simulink model "WF_offshore"  (R2024a)
settings: Solver=VariableStepAuto  StartTime=0  StopTime=1  RelTol=1e-3
values from neighbouring files (symbols this model uses):
  WF = calculate_WF(WF)    [WF_parameter_variation.m]
undefined symbols (not defined in the file or in its folder): L, Lg, R
libraries: spsSeriesRLCBranchLib x24, spsGroundLib x11, simulink_extras x8, spsThreePhaseVIMeasurementLib x6, spsControlledVoltageSourceLib x6, spsIdealSwitchLib x6, simulink x4, spsVariableInductorLib x3, spsThreePhaseSeriesRLCBranchLib x2, spsThreePhaseTransformerTwoWindingsLib x2, powerlib_extras x1, spspowerguiLib x1
(part 1 of 2)
settings Model: Creator=andrsmit  LastModifiedBy=andrsmit
settings DataIOCC: InitialState=op.xFinal  SaveFinalState=on  SaveOperatingPoint=on

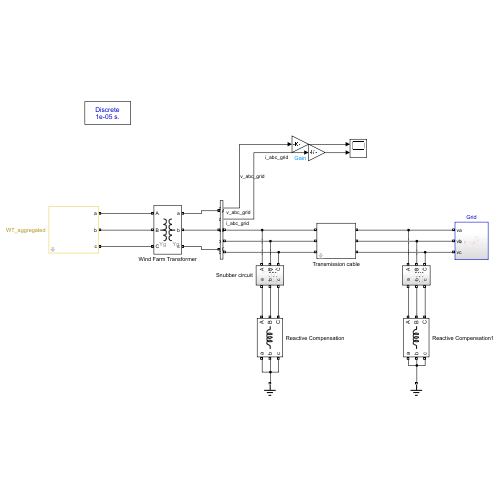
[thumbnail: Simulink's stored preview of the top-level diagram]
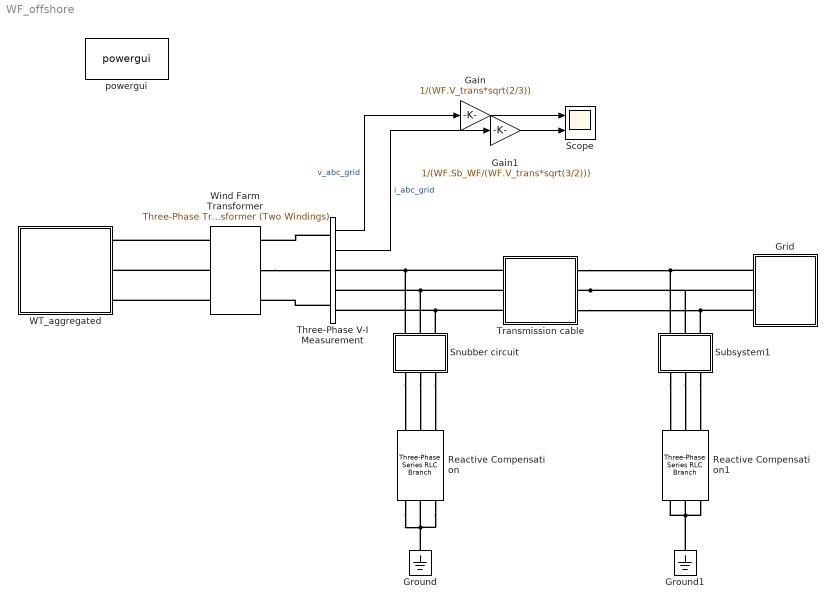
== system WF_offshore ==
  Gain : Gain  Gain=1/(WF.V_trans*sqrt(2/3))
  Gain1 : Gain  Gain=1/(WF.Sb_WF/(WF.V_trans*sqrt(3/2)))
  Grid : Subsystem
  Ground : spsGroundLib/Ground  LConnTagsString=a
  Ground1 : spsGroundLib/Ground  LConnTagsString=a
  Reactive Compensation : spsThreePhaseSeriesRLCBranchLib/Three-Phase Series RLC Branch  LConnTagsString=A|B|C  RConnTagsString=A|B|C  BranchType=L  Resistance=100  Inductance=WF.L_comp  Capacitance=1e-6  Measurements=None
  Reactive Compensation1 : spsThreePhaseSeriesRLCBranchLib/Three-Phase Series RLC Branch  LConnTagsString=A|B|C  RConnTagsString=A|B|C  BranchType=L  Resistance=100  Inductance=WF.L_comp  Capacitance=1e-6  Measurements=None
  Scope : Scope  NumInputPorts=2
  Snubber circuit : Subsystem
  Subsystem1 : Subsystem
  Three-Phase V-I Measurement : spsThreePhaseVIMeasurementLib/Three-Phase V-I Measurement  VoltageMeasurement=phase-to-ground  SetLabelV=off  LabelV=Vabc  Vpu=off  VpuLL=off  CurrentMeasurement=yes  SetLabelI=off  LabelI=Iabc  Ipu=off  Pbase=100e6  Vbase=500e3  OutputType=Complex  PhasorSimulation=off  PSBequivalent=0
  Transmission cable : Subsystem  mask{D=WF.Trans.D_C, r=WF.Trans.r_c_eff, l=WF.Trans.l_c_eff, c=WF.Trans.c_c_eff}
      mask prompts: D "Distance (km)"; r "Resistance/km (Ohms/km)"; l "Inductance/km (H/km)"; c "Capacitance/km (F/km)"
      mask DialogControl DescTextVar Prompt: Single PI-line cable model, with no coupling/connection between phases
  WT_aggregated : Subsystem  mask{cvtr=WF.WT.cvtr_agg}
      mask prompts: cvtr "converter name"
  Wind Farm Transformer : spsThreePhaseTransformerTwoWindingsLib/Three-Phase Transformer (Two Windings)  Winding1Connection=Yg  Winding2Connection=Yg  CoreType=Three single-phase transformers  SetSaturation=off  Hysteresis=off  DataFile='hysteresis'  SetInitialFlux=off  Measurements=None  UNITS=pu  NominalPower=[WF.Sb_WF , WF.f1]  Winding1=[WF.V_coll , WF.r_tf/2, WF.l_tf/2]  Winding2=[WF.V_trans, WF.r_tf/2, WF.l_tf/2]  Rm=5000  Lm=0  L0=0.5  Saturation=[ 0,0 ; 0.0024,1.2 ; 1.0,1.52 ]  InitialFluxes=[ 0.8 , -0.8 , 0.7 ]  BreakLoop=off  DiscreteSolver=Trapezoidal iterative  DataType=off  TransfoNumber=1
  powergui : spspowerguiLib/powergui  Priority=2  SimulationMode=Discrete  SampleTime=WF.WT.cvtr_agg.parameters.Ts  frequency=60  Iterations=50  frequencyindice=0  Pbase=100e6  ErrMax=0.0001  UnitsV=kV  UnitsW=MW  buscounter=0  FunctionMessages=off  echomessages=off  EnableUseOfTLC=off  CurrentSourceSwitches=off  DisableSnubberDevices=off  DisableRonSwitches=off  DisableVfSwitches=off  DisplayEquations=off  AutomaticDiscreteSolvers=off  SolverType=Tustin  Interpol=off  ExternalGateDelay=off  methode=off  Ts=0  x0status=blocks  SPID=off  SwTol=0  HookPort=off  NonlinearTolerance=1e-4  nMaxIteration=100  ContinueOnMaxIteration=off  RestoreLinks=warning  ResistiveCurrentMeasurement=off  Frange=logspace(0,3,50)  Ylog=off  Xlog=off  ShowGrid=off  save=off  variable=ZData  structure=0  ZoomFFT=on  StartTime=0.0  cycles=1  DisplayStyle=1  fundamental=60  FreqAxis=off  MaxFrequency=1000  frequencyindicesteady=1  RmsSteady=1  display=off
  wires:
  Three-Phase V-I Measurement/1 -> Gain/1  "v_abc_grid"
  Three-Phase V-I Measurement/2 -> Gain1/1  "i_abc_grid"
  Gain1/1 -> Scope/2
  Gain/1 -> Scope/1
  connections:
  Three-Phase V-I Measurement/LConn1 -- Wind Farm Transformer/RConn1
  Wind Farm Transformer/RConn2 -- Three-Phase V-I Measurement/LConn2
  Three-Phase V-I Measurement/LConn3 -- Wind Farm Transformer/RConn3
  Transmission cable/RConn1 -- Grid/RConn1 -- Subsystem1/LConn1
  Transmission cable/RConn2 -- Grid/RConn2 -- Subsystem1/LConn2
  Transmission cable/LConn3 -- Snubber circuit/LConn3 -- Three-Phase V-I Measurement/RConn3
  Ground/LConn1 -- Reactive Compensation/RConn1 -- Reactive Compensation/RConn3 -- Reactive Compensation/RConn2
  Reactive Compensation1/RConn3 -- Reactive Compensation1/RConn1 -- Ground1/LConn1 -- Reactive Compensation1/RConn2
  Transmission cable/RConn3 -- Grid/RConn3 -- Subsystem1/LConn3
  Snubber circuit/RConn2 -- Reactive Compensation/LConn2
  Snubber circuit/RConn1 -- Reactive Compensation/LConn1
  Transmission cable/LConn2 -- Snubber circuit/LConn2 -- Three-Phase V-I Measurement/RConn2
  Snubber circuit/RConn3 -- Reactive Compensation/LConn3
  Transmission cable/LConn1 -- Three-Phase V-I Measurement/RConn1 -- Snubber circuit/LConn1
  Subsystem1/RConn3 -- Reactive Compensation1/LConn3
  Subsystem1/RConn1 -- Reactive Compensation1/LConn1
  Subsystem1/RConn2 -- Reactive Compensation1/LConn2
  Wind Farm Transformer/LConn3 -- WT_aggregated/RConn3
  Wind Farm Transformer/LConn2 -- WT_aggregated/RConn2
  Wind Farm Transformer/LConn1 -- WT_aggregated/RConn1

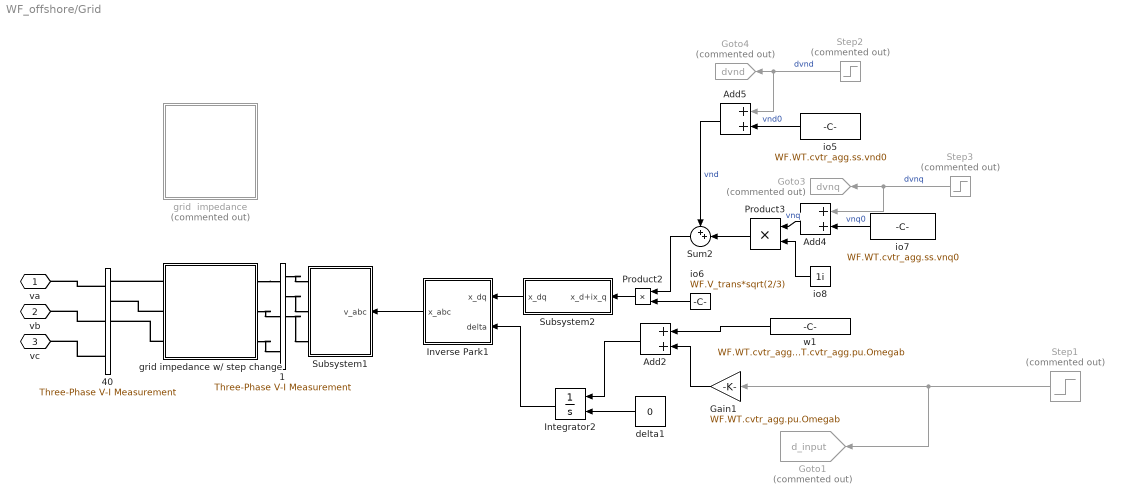
== system WF_offshore/Grid ==
  1 : spsThreePhaseVIMeasurementLib/Three-Phase V-I Measurement  VoltageMeasurement=phase-to-ground  SetLabelV=off  LabelV=Vabc_1  Vpu=off  VpuLL=off  CurrentMeasurement=yes  SetLabelI=off  LabelI=Iabc_1  Ipu=off  Pbase=100e6  Vbase=Bus(1,2)*1e3  OutputType=Complex  PhasorSimulation=off  PSBequivalent=0
  40 : spsThreePhaseVIMeasurementLib/Three-Phase V-I Measurement  VoltageMeasurement=phase-to-ground  SetLabelV=off  LabelV=Vabc_1  Vpu=off  VpuLL=off  CurrentMeasurement=yes  SetLabelI=off  LabelI=Iabc_1  Ipu=off  Pbase=100e6  Vbase=Bus(1,2)*1e3  OutputType=Complex  PhasorSimulation=off  PSBequivalent=0
  Add2 : Sum
  Add4 : Sum
  Add5 : Sum
  Gain1 : Gain  Gain=WF.WT.cvtr_agg.pu.Omegab
  Goto1 : Goto  Commented=on  GotoTag=d_input  TagVisibility=global
  Goto3 : Goto  Commented=on  GotoTag=dvnq  TagVisibility=global
  Goto4 : Goto  Commented=on  GotoTag=dvnd  TagVisibility=global
  Integrator2 : Integrator  InitialConditionSource=external
  Inverse Park1 : Subsystem
  Product2 : Product
  Product3 : Product
  Step1 : Step  Commented=on  Time=0.1  After=1e-4  SampleTime=0
  Step2 : Step  Commented=on  Time=0.1  After=0.01  SampleTime=0
  Step3 : Step  Commented=on  Time=0.1  After=0.01  SampleTime=0
  Subsystem1 : Subsystem
  Subsystem2 : Subsystem
  Sum2 : Sum  Inputs=++|
  delta1 : Constant  Value=0
  grid  impedance : Subsystem  Commented=on
  grid impedance w/ step change : Subsystem
  io5 : Constant  Value=WF.WT.cvtr_agg.ss.vnd0
  io6 : Constant  Value=WF.V_trans*sqrt(2/3)
  io7 : Constant  Value=WF.WT.cvtr_agg.ss.vnq0
  io8 : Constant  Value=1i
  w1 : Constant  Value=WF.WT.cvtr_agg.parameters.Omegag*WF.WT.cvtr_agg.pu.Omegab
  va : PMIOPort  Side=Right
  vb : PMIOPort  Port=2  Side=Right
  vc : PMIOPort  Port=3  Side=Right
  wires:
  Integrator2/1 -> Inverse Park1/2(delta)
  io5/1 -> Add5/2  "vnd0"
  Add4/1 -> Product3/1  "vnq"
  Subsystem2/1(x_dq) -> Inverse Park1/1(x_dq)
  Add2/1 -> Integrator2/1
  Inverse Park1/1(x_abc) -> Subsystem1/1(v_abc)
  Sum2/1 -> Product2/1
  io7/1 -> Add4/2  "vnq0"
  w1/1 -> Add2/1
  Step1/1 -> Goto1/1, Gain1/1
  Step3/1 -> Goto3/1, Add4/1  "dvnq"
  Add5/1 -> Sum2/1  "vnd"
  delta1/1 -> Integrator2/2
  Step2/1 -> Add5/1, Goto4/1  "dvnd"
  Product2/1 -> Subsystem2/1(x_d+ix_q)
  io8/1 -> Product3/2
  io6/1 -> Product2/2
  Product3/1 -> Sum2/2
  Gain1/1 -> Add2/2
  connections:
  40/LConn1 -- vc/RConn1
  40/LConn2 -- vb/RConn1
  40/LConn3 -- va/RConn1
  grid impedance w/ step change/LConn1 -- 40/RConn3
  grid impedance w/ step change/LConn2 -- 40/RConn2
  grid impedance w/ step change/LConn3 -- 40/RConn1
  grid impedance w/ step change/RConn1 -- 1/LConn3
  grid impedance w/ step change/RConn2 -- 1/LConn2
  grid impedance w/ step change/RConn3 -- 1/LConn1
  1/RConn3 -- Subsystem1/RConn1
  1/RConn2 -- Subsystem1/RConn2
  1/RConn1 -- Subsystem1/RConn3

== system WF_offshore/Snubber circuit ==
  Ideal Switch : spsIdealSwitchLib/Ideal Switch  Ron=WF.R_comp  Lon=0  IC=0  Rs=WF.r_diss*WF.Imp.Z_b_G  Cs=inf  Measurements=off
  Ideal Switch1 : spsIdealSwitchLib/Ideal Switch  Ron=WF.R_comp  Lon=0  IC=0  Rs=WF.r_diss*WF.Imp.Z_b_G  Cs=inf  Measurements=off
  Ideal Switch2 : spsIdealSwitchLib/Ideal Switch  Ron=WF.R_comp  Lon=0  IC=0  Rs=WF.r_diss*WF.Imp.Z_b_G  Cs=inf  Measurements=off
  Step : Step  Time=0.5  SampleTime=0
  " A" : PMIOPort  Side=Left
  " B" : PMIOPort  Port=2  Side=Left
  " C" : PMIOPort  Port=3  Side=Left
  "  a" : PMIOPort  Port=4  Side=Right
  "  b" : PMIOPort  Port=5  Side=Right
  "  c" : PMIOPort  Port=6  Side=Right
  wires:
  Step/1 -> Ideal Switch2/1, Ideal Switch1/1, Ideal Switch/1
  connections:
  "  a"/RConn1 -- Ideal Switch/RConn1
  Ideal Switch2/LConn1 -- " C"/RConn1
  Ideal Switch2/RConn1 -- "  c"/RConn1
  " A"/RConn1 -- Ideal Switch/LConn1
  Ideal Switch1/RConn1 -- "  b"/RConn1
  Ideal Switch1/LConn1 -- " B"/RConn1

== system WF_offshore/Subsystem1 ==
  Ideal Switch : spsIdealSwitchLib/Ideal Switch  Ron=WF.R_comp  Lon=0  IC=0  Rs=WF.r_diss*WF.Imp.Z_b_G  Cs=inf  Measurements=off
  Ideal Switch1 : spsIdealSwitchLib/Ideal Switch  Ron=WF.R_comp  Lon=0  IC=0  Rs=WF.r_diss*WF.Imp.Z_b_G  Cs=inf  Measurements=off
  Ideal Switch2 : spsIdealSwitchLib/Ideal Switch  Ron=WF.R_comp  Lon=0  IC=0  Rs=WF.r_diss*WF.Imp.Z_b_G  Cs=inf  Measurements=off
  Step : Step  Time=0.5  SampleTime=0
  " A" : PMIOPort  Side=Left
  " B" : PMIOPort  Port=2  Side=Left
  " C" : PMIOPort  Port=3  Side=Left
  "  a" : PMIOPort  Port=4  Side=Right
  "  b" : PMIOPort  Port=5  Side=Right
  "  c" : PMIOPort  Port=6  Side=Right
  wires:
  Step/1 -> Ideal Switch2/1, Ideal Switch1/1, Ideal Switch/1
  connections:
  "  a"/RConn1 -- Ideal Switch/RConn1
  Ideal Switch2/LConn1 -- " C"/RConn1
  Ideal Switch2/RConn1 -- "  c"/RConn1
  " A"/RConn1 -- Ideal Switch/LConn1
  Ideal Switch1/RConn1 -- "  b"/RConn1
  Ideal Switch1/LConn1 -- " B"/RConn1

== system WF_offshore/Transmission cable ==
  Subsystem : Subsystem
  Subsystem1 : Subsystem
  Subsystem2 : Subsystem
  A : PMIOPort  Side=Left
  a : PMIOPort  Port=2  Side=Right
  B : PMIOPort  Port=3  Side=Left
  b : PMIOPort  Port=4  Side=Right
  C : PMIOPort  Port=5  Side=Left
  c : PMIOPort  Port=6  Side=Right
  connections:
  Subsystem/RConn1 -- a/RConn1
  Subsystem/LConn1 -- A/RConn1
  Subsystem1/LConn1 -- B/RConn1
  Subsystem2/RConn1 -- c/RConn1
  Subsystem1/RConn1 -- b/RConn1
  Subsystem2/LConn1 -- C/RConn1

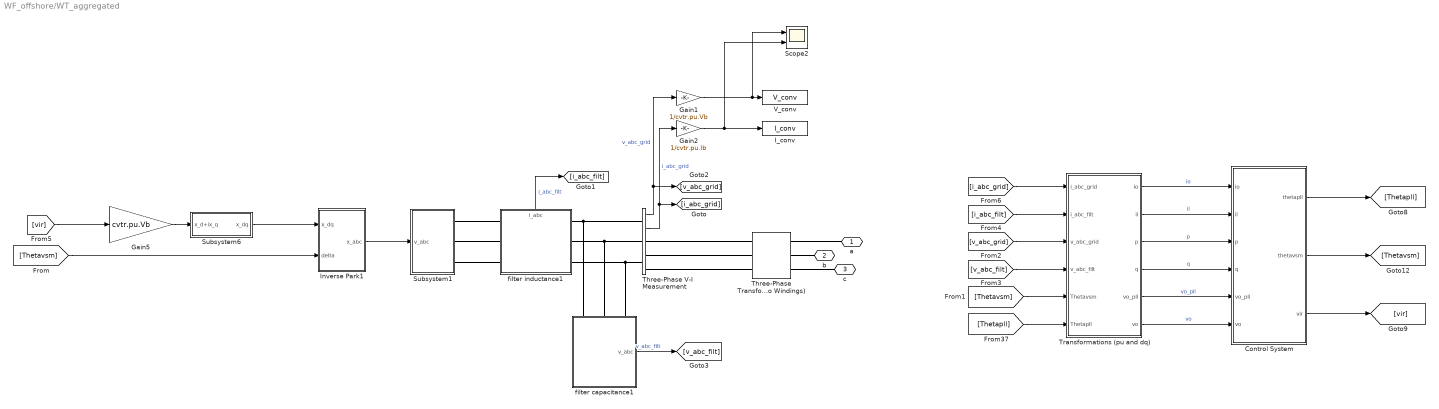
== system WF_offshore/WT_aggregated ==
  Control System : Subsystem  mask{Ts_control=cvtr.parameters.T_cont}
      mask prompts: Ts_control "Sample Time"
  Gain1 : Gain  Gain=1/cvtr.pu.Vb
  Gain2 : Gain  Gain=1/cvtr.pu.Ib
  Gain5 : Gain  Gain=cvtr.pu.Vb
  I_conv : ToWorkspace  VariableName=I_conv  SaveFormat=Structure With Time  SampleTime=-1
      settings: MaxDataPoints=1000000
  Inverse Park1 : Subsystem
  Scope2 : Scope  NumInputPorts=2
  Subsystem1 : Subsystem
  Subsystem6 : Subsystem
  Three-Phase Transformer (Two Windings) : spsThreePhaseTransformerTwoWindingsLib/Three-Phase Transformer (Two Windings)  Winding1Connection=Yg  Winding2Connection=Yg  CoreType=Three single-phase transformers  SetSaturation=off  Hysteresis=off  DataFile='hysteresis'  SetInitialFlux=off  Measurements=None  UNITS=pu  NominalPower=[WF.Sb_WF , WF.f1 ]  Winding1=[WF.WT.V_wt ,WF.WT.r_tf/2 , WF.WT.l_tf/2]  Winding2=[WF.V_coll , WF.WT.r_tf/2, WF.WT.l_tf/2]  Rm=5000  Lm=0  L0=0.5  Saturation=[ 0,0 ; 0.0024,1.2 ; 1.0,1.52 ]  InitialFluxes=[ 0.8 , -0.8 , 0.7 ]  BreakLoop=off  DiscreteSolver=Trapezoidal iterative  DataType=off  TransfoNumber=1
  Three-Phase V-I Measurement : spsThreePhaseVIMeasurementLib/Three-Phase V-I Measurement  VoltageMeasurement=phase-to-ground  SetLabelV=off  LabelV=Vabc  Vpu=off  VpuLL=off  CurrentMeasurement=yes  SetLabelI=off  LabelI=Iabc  Ipu=off  Pbase=100e6  Vbase=500e3  OutputType=Complex  PhasorSimulation=off  PSBequivalent=0
  Transformations (pu and dq) : Subsystem
  V_conv : ToWorkspace  VariableName=V_conv  SaveFormat=Structure With Time  SampleTime=-1
      settings: MaxDataPoints=1000000
  filter capacitance1 : Subsystem
      settings: PortSchema="{\"entries\":[{\"content\":{\"sides\":[{\"content\":{\"connectorIds\":[\"LConn1\",\"LConn2\",\"LConn3\"]},\"type\":\"ConnectorPlacement.EquallySpacedRectSide\",\"uuid\":\"e81be3d5-6303-4565-8ca3-afc618f21d70\"},{\"content\":{\"connectorIds\":[],\"side\":\"RIGHT\"},\"type\":\"ConnectorPlacement.EquallySpacedRectSide\",\"uuid\":\"458d9030-e614-487d-87de-3e53be7c7da4\"},{\"content\":{\"connectorIds\":[],\"side\":\"TOP\"},\"type\":\"ConnectorPlacement.EquallySpacedRectSide\",\"uuid\":\"a29d66a0-f095-498d-bb9b-96c7f47699d3\"},{\"content\":{\"connectorIds\":[\"Out1\"],\"side\":\"BOTTOM\"},\"type\":\"ConnectorPlacement.EquallySpacedRectSide\",\"uuid\":\"afc68874-c098-43f5-9b37-53a3b484513b\"}]},\"type\":\"ConnectorPlacement.EquallySpacedConnector\",\"uuid\":\"37f495dd-1c12-4bb8-af72-7ef46bbd951c\"}],\"packageUris\":[\"http://schema.mathworks.com/mf0/Connector/R2020b\"],\"version\":\"1.0\"}"
  filter inductance1 : Subsystem
      settings: PortSchema="{\"entries\":[{\"content\":{\"sides\":[{\"content\":{\"connectorIds\":[\"LConn1\",\"LConn2\",\"LConn3\"]},\"type\":\"ConnectorPlacement.EquallySpacedRectSide\",\"uuid\":\"d3d60048-9578-4fa3-8d11-9c8a66a4b1f9\"},{\"content\":{\"connectorIds\":[\"RConn1\",\"RConn2\",\"RConn3\"],\"side\":\"RIGHT\"},\"type\":\"ConnectorPlacement.EquallySpacedRectSide\",\"uuid\":\"184a2c1d-36ab-46d1-99e4-db01aa31ec94\"},{\"content\":{\"connectorIds\":[\"Out1\"],\"side\":\"TOP\"},\"type\":\"ConnectorPlacement.EquallySpacedRectSide\",\"uuid\":\"db651021-9d7f-4124-8d21-ede853163467\"}]},\"type\":\"ConnectorPlacement.EquallySpacedConnector\",\"uuid\":\"723d0964-19fd-4dbe-91e3-e4ea0bb1cca9\"}],\"packageUris\":[\"http://schema.mathworks.com/mf0/Connector/R2020b\"],\"version\":\"1.0\"}"
  a : PMIOPort  Side=Right
  b : PMIOPort  Port=2  Side=Right
  c : PMIOPort  Port=3  Side=Right
  wires:
  Control System/2(thetavsm) -> [Thetavsm]
  Control System/3(vir) -> [vir]
  Control System/1(thetapll) -> [Thetapll]
  Transformations (pu and dq)/2(il) -> Control System/2(il)  "il"
  Transformations (pu and dq)/1(io) -> Control System/1(io)  "io"
  Transformations (pu and dq)/3(p) -> Control System/3(p)  "p"
  Transformations (pu and dq)/4(q) -> Control System/4(q)  "q"
  Transformations (pu and dq)/5(vo_pll) -> Control System/5(vo_pll)  "vo_pll"
  Transformations (pu and dq)/6(vo) -> Control System/6(vo)  "vo"
  [Thetavsm] -> Transformations (pu and dq)/5(Thetavsm)
  [Thetapll] -> Transformations (pu and dq)/6(Thetapll)
  [vir] -> Gain5/1
  Subsystem6/1(x_dq) -> Inverse Park1/1(x_dq)
  Gain5/1 -> Subsystem6/1(x_d+ix_q)
  Three-Phase V-I Measurement/2 -> Gain2/1, [i_abc_grid]  "i_abc_grid"
  Inverse Park1/1(x_abc) -> Subsystem1/1(v_abc)
  Three-Phase V-I Measurement/1 -> Gain1/1, [v_abc_grid]  "v_abc_grid"
  [Thetavsm] -> Inverse Park1/2(delta)
  filter capacitance1/1(v_abc) -> [v_abc_filt]  "v_abc_filt"
  filter inductance1/1(i_abc) -> [i_abc_filt]  "i_abc_filt"
  [v_abc_grid] -> Transformations (pu and dq)/3(v_abc_grid)
  [v_abc_filt] -> Transformations (pu and dq)/4(v_abc_filt)
  [i_abc_filt] -> Transformations (pu and dq)/2(i_abc_filt)
  [i_abc_grid] -> Transformations (pu and dq)/1(i_abc_grid)
  Gain1/1 -> Scope2/1, V_conv/1
  Gain2/1 -> Scope2/2, I_conv/1
  connections:
  filter inductance1/RConn3 -- filter capacitance1/LConn3 -- Three-Phase V-I Measurement/LConn3
  filter inductance1/RConn1 -- filter capacitance1/LConn1 -- Three-Phase V-I Measurement/LConn1
  filter inductance1/RConn2 -- filter capacitance1/LConn2 -- Three-Phase V-I Measurement/LConn2
  Subsystem1/RConn1 -- filter inductance1/LConn1
  Subsystem1/RConn2 -- filter inductance1/LConn2
  Subsystem1/RConn3 -- filter inductance1/LConn3
  Three-Phase Transformer (Two Windings)/RConn1 -- a/RConn1
  Three-Phase Transformer (Two Windings)/RConn2 -- b/RConn1
  Three-Phase Transformer (Two Windings)/RConn3 -- c/RConn1
  Three-Phase Transformer (Two Windings)/LConn1 -- Three-Phase V-I Measurement/RConn1
  Three-Phase Transformer (Two Windings)/LConn2 -- Three-Phase V-I Measurement/RConn2
  Three-Phase Transformer (Two Windings)/LConn3 -- Three-Phase V-I Measurement/RConn3

== system WF_offshore/Grid/Inverse Park1 ==
  x_dq : Inport
  delta : Inport  Port=2
  Demux1 : Demux  Outputs=2
  Fcn : Fcn  Expr=cos(u(3))*u(1)-sin(u(3))*u(2)
  Fcn1 : Fcn  Expr=cos(u(3)-2/3*pi)*u(1)-sin(u(3)-2/3*pi)*u(2)
  Fcn2 : Fcn  Expr=cos(u(3)+2/3*pi)*u(1)-sin(u(3)+2/3*pi)*u(2)
  Mux : Mux  Inputs=3
  Mux1 : Mux  Inputs=3
  x_abc : Outport
  wires:
  Mux1/1 -> x_abc/1
  Mux/1 -> Fcn1/1, Fcn2/1, Fcn/1
  delta/1 -> Mux/3
  x_dq/1 -> Demux1/1
  Demux1/2 -> Mux/2
  Demux1/1 -> Mux/1
  Fcn/1 -> Mux1/1
  Fcn1/1 -> Mux1/2
  Fcn2/1 -> Mux1/3

== system WF_offshore/Grid/Subsystem1 ==
  v_abc : Inport
  Controlled Voltage Source : spsControlledVoltageSourceLib/Controlled Voltage Source  Initialize=on  Source_Type=AC  Amplitude=0  Phase=0  Frequency=0  Measurements=None
  Controlled Voltage Source1 : spsControlledVoltageSourceLib/Controlled Voltage Source  Initialize=on  Source_Type=AC  Amplitude=0  Phase=0  Frequency=0  Measurements=None
  Controlled Voltage Source2 : spsControlledVoltageSourceLib/Controlled Voltage Source  Initialize=on  Source_Type=AC  Amplitude=0  Phase=0  Frequency=0  Measurements=None
  Demux : Demux  Outputs=3
  Ground1 : spsGroundLib/Ground  LConnTagsString=a
  va : PMIOPort  Side=Right
  vb : PMIOPort  Port=2  Side=Right
  vc : PMIOPort  Port=3  Side=Right
  wires:
  Demux/1 -> Controlled Voltage Source/1
  Demux/2 -> Controlled Voltage Source1/1
  Demux/3 -> Controlled Voltage Source2/1
  v_abc/1 -> Demux/1
  connections:
  Controlled Voltage Source2/LConn1 -- Ground1/LConn1 -- Controlled Voltage Source1/LConn1 -- Controlled Voltage Source/LConn1
  va/RConn1 -- Controlled Voltage Source/RConn1
  vb/RConn1 -- Controlled Voltage Source1/RConn1
  vc/RConn1 -- Controlled Voltage Source2/RConn1

== system WF_offshore/Grid/Subsystem2 ==
  x_d+ix_q : Inport
  Complex to Real-Imag2 : ComplexToRealImag
  Mux : Mux  Inputs=2
  x_dq : Outport
  wires:
  Complex to Real-Imag2/1 -> Mux/1
  Complex to Real-Imag2/2 -> Mux/2
  Mux/1 -> x_dq/1
  x_d+ix_q/1 -> Complex to Real-Imag2/1

== system WF_offshore/Grid/grid  impedance ==
  Series RLC Branch : spsSeriesRLCBranchLib/Series RLC Branch  LConnTagsString=__new0  RConnTagsString=__new0  BranchType=RL  Resistance=(WF.Trans.rg)*WF.Imp.Z_b_G  Inductance=(WF.Trans.lg)*(WF.Imp.Z_b_G/(2*pi*WF.f1))  SetiL0=off  InitialCurrent=cvtr.ss.io0a  Capacitance=1e-6  Setx0=off  InitialVoltage=0  Measurements=None
  Series RLC Branch1 : spsSeriesRLCBranchLib/Series RLC Branch  LConnTagsString=__new0  RConnTagsString=__new0  BranchType=RL  Resistance=(WF.Trans.rg)*WF.Imp.Z_b_G  Inductance=(WF.Trans.lg)*(WF.Imp.Z_b_G/(2*pi*WF.f1))  SetiL0=off  InitialCurrent=cvtr.ss.io0b  Capacitance=1e-6  Setx0=off  InitialVoltage=0  Measurements=None
  Series RLC Branch2 : spsSeriesRLCBranchLib/Series RLC Branch  LConnTagsString=__new0  RConnTagsString=__new0  BranchType=RL  Resistance=(WF.Trans.rg)*WF.Imp.Z_b_G  Inductance=(WF.Trans.lg)*(WF.Imp.Z_b_G/(2*pi*WF.f1))  SetiL0=off  InitialCurrent=cvtr.ss.io0c  Capacitance=1e-6  Setx0=off  InitialVoltage=0  Measurements=None
  A : PMIOPort  Side=Left
  a : PMIOPort  Port=2  Side=Right
  B : PMIOPort  Port=3  Side=Left
  b : PMIOPort  Port=4  Side=Right
  C : PMIOPort  Port=5  Side=Left
  c : PMIOPort  Port=6  Side=Right
  connections:
  Series RLC Branch/RConn1 -- a/RConn1
  Series RLC Branch1/RConn1 -- b/RConn1
  Series RLC Branch2/RConn1 -- c/RConn1
  A/RConn1 -- Series RLC Branch/LConn1
  B/RConn1 -- Series RLC Branch1/LConn1
  C/RConn1 -- Series RLC Branch2/LConn1

== system WF_offshore/Grid/grid impedance w// step change ==
  Rate Limiter : RateLimiter  SampleTimeMode=inherited
  Series RLC Branch : spsSeriesRLCBranchLib/Series RLC Branch  LConnTagsString=__new0  RConnTagsString=__new0  BranchType=R  Resistance=(WF.Trans.rg)*WF.Imp.Z_b_G  Inductance=Lg  SetiL0=off  InitialCurrent=cvtr.ss.io0a  Capacitance=1e-6  Setx0=off  InitialVoltage=0  Measurements=None
  Series RLC Branch1 : spsSeriesRLCBranchLib/Series RLC Branch  LConnTagsString=__new0  RConnTagsString=__new0  BranchType=R  Resistance=(WF.Trans.rg)*WF.Imp.Z_b_G  Inductance=Lg  SetiL0=off  InitialCurrent=cvtr.ss.io0b  Capacitance=1e-6  Setx0=off  InitialVoltage=0  Measurements=None
  Series RLC Branch2 : spsSeriesRLCBranchLib/Series RLC Branch  LConnTagsString=__new0  RConnTagsString=__new0  BranchType=R  Resistance=(WF.Trans.rg)*WF.Imp.Z_b_G  Inductance=Lg  SetiL0=off  InitialCurrent=cvtr.ss.io0c  Capacitance=1e-6  Setx0=off  InitialVoltage=0  Measurements=None
  Series RLC Branch3 : spsSeriesRLCBranchLib/Series RLC Branch  LConnTagsString=__new0  RConnTagsString=__new0  BranchType=R  Resistance=1e9  Inductance=Lg  SetiL0=off  InitialCurrent=cvtr.ss.io0a  Capacitance=1e-6  Setx0=off  InitialVoltage=0  Measurements=None
  Series RLC Branch4 : spsSeriesRLCBranchLib/Series RLC Branch  LConnTagsString=__new0  RConnTagsString=__new0  BranchType=R  Resistance=1e9  Inductance=Lg  SetiL0=off  InitialCurrent=cvtr.ss.io0a  Capacitance=1e-6  Setx0=off  InitialVoltage=0  Measurements=None
  Series RLC Branch5 : spsSeriesRLCBranchLib/Series RLC Branch  LConnTagsString=__new0  RConnTagsString=__new0  BranchType=R  Resistance=1e9  Inductance=Lg  SetiL0=off  InitialCurrent=cvtr.ss.io0a  Capacitance=1e-6  Setx0=off  InitialVoltage=0  Measurements=None
  Step : Step  Time=0.2  Before=WF.Trans.lg*0.5*(WF.Imp.Z_b_G/(2*pi*WF.f1))  After=WF.Trans.lg*(WF.Imp.Z_b_G/(2*pi*WF.f1))  SampleTime=0
  Variable Inductor : spsVariableInductorLib/Variable Inductor  methode=Backward Euler  Labsmin=1e-6  Initialize=off  iL0=0  L0=1e-3  Vl0=0
      settings: LibrarySourceBlock=sps_lib/Passives/Variable Inductor
  Variable Inductor1 : spsVariableInductorLib/Variable Inductor  methode=Backward Euler  Labsmin=1e-6  Initialize=off  iL0=0  L0=1e-3  Vl0=0
      settings: LibrarySourceBlock=sps_lib/Passives/Variable Inductor
  Variable Inductor2 : spsVariableInductorLib/Variable Inductor  methode=Backward Euler  Labsmin=1e-6  Initialize=off  iL0=0  L0=1e-3  Vl0=0
      settings: LibrarySourceBlock=sps_lib/Passives/Variable Inductor
  A : PMIOPort  Side=Left
  a : PMIOPort  Port=2  Side=Right
  B : PMIOPort  Port=3  Side=Left
  b : PMIOPort  Port=4  Side=Right
  C : PMIOPort  Port=5  Side=Left
  c : PMIOPort  Port=6  Side=Right
  wires:
  Step/1 -> Rate Limiter/1
  Rate Limiter/1 -> Variable Inductor2/1, Variable Inductor1/1, Variable Inductor/1
  connections:
  Series RLC Branch2/RConn1 -- c/RConn1
  Series RLC Branch1/RConn1 -- b/RConn1
  Series RLC Branch/RConn1 -- a/RConn1
  Series RLC Branch/LConn1 -- Series RLC Branch5/RConn1 -- Variable Inductor/RConn1
  Series RLC Branch1/LConn1 -- Series RLC Branch4/RConn1 -- Variable Inductor1/RConn1
  Series RLC Branch2/LConn1 -- Series RLC Branch3/RConn1 -- Variable Inductor2/RConn1
  A/RConn1 -- Series RLC Branch5/LConn1 -- Variable Inductor/LConn1
  B/RConn1 -- Series RLC Branch4/LConn1 -- Variable Inductor1/LConn1
  C/RConn1 -- Series RLC Branch3/LConn1 -- Variable Inductor2/LConn1

== system WF_offshore/Transmission cable/Subsystem ==
  Ground : spsGroundLib/Ground  LConnTagsString=a
  Ground1 : spsGroundLib/Ground  LConnTagsString=a
  Series RLC Branch : spsSeriesRLCBranchLib/Series RLC Branch  LConnTagsString=__new0  RConnTagsString=__new0  BranchType=C  Resistance=1  Inductance=1e-3  SetiL0=off  InitialCurrent=0  Capacitance=c/2*D  Setx0=off  InitialVoltage=0  Measurements=None
  Series RLC Branch1 : spsSeriesRLCBranchLib/Series RLC Branch  LConnTagsString=__new0  RConnTagsString=__new0  BranchType=RL  Resistance=r*D  Inductance=l*D  SetiL0=off  InitialCurrent=0  Capacitance=1e-6  Setx0=off  InitialVoltage=0  Measurements=None
  Series RLC Branch2 : spsSeriesRLCBranchLib/Series RLC Branch  LConnTagsString=__new0  RConnTagsString=__new0  BranchType=C  Resistance=1  Inductance=1e-3  SetiL0=off  InitialCurrent=0  Capacitance=c/2*D  Setx0=off  InitialVoltage=0  Measurements=None
  Conn1 : PMIOPort  Side=Left
  Conn2 : PMIOPort  Port=2  Side=Right
  connections:
  Series RLC Branch/LConn1 -- Conn1/RConn1 -- Series RLC Branch1/RConn1
  Ground1/LConn1 -- Series RLC Branch2/RConn1
  Ground/LConn1 -- Series RLC Branch/RConn1
  Series RLC Branch1/LConn1 -- Conn2/RConn1 -- Series RLC Branch2/LConn1

== system WF_offshore/Transmission cable/Subsystem1 ==
  Ground : spsGroundLib/Ground  LConnTagsString=a
  Ground1 : spsGroundLib/Ground  LConnTagsString=a
  Series RLC Branch : spsSeriesRLCBranchLib/Series RLC Branch  LConnTagsString=__new0  RConnTagsString=__new0  BranchType=C  Resistance=1  Inductance=1e-3  SetiL0=off  InitialCurrent=0  Capacitance=c/2*D  Setx0=off  InitialVoltage=0  Measurements=None
  Series RLC Branch1 : spsSeriesRLCBranchLib/Series RLC Branch  LConnTagsString=__new0  RConnTagsString=__new0  BranchType=RL  Resistance=r*D  Inductance=l*D  SetiL0=off  InitialCurrent=0  Capacitance=1e-6  Setx0=off  InitialVoltage=0  Measurements=None
  Series RLC Branch2 : spsSeriesRLCBranchLib/Series RLC Branch  LConnTagsString=__new0  RConnTagsString=__new0  BranchType=C  Resistance=1  Inductance=1e-3  SetiL0=off  InitialCurrent=0  Capacitance=c/2*D  Setx0=off  InitialVoltage=0  Measurements=None
  Conn1 : PMIOPort  Side=Left
  Conn2 : PMIOPort  Port=2  Side=Right
  connections:
  Series RLC Branch2/LConn1 -- Conn2/RConn1 -- Series RLC Branch1/LConn1
  Ground/LConn1 -- Series RLC Branch/RConn1
  Ground1/LConn1 -- Series RLC Branch2/RConn1
  Series RLC Branch1/RConn1 -- Conn1/RConn1 -- Series RLC Branch/LConn1

== system WF_offshore/Transmission cable/Subsystem2 ==
  Ground : spsGroundLib/Ground  LConnTagsString=a
  Ground1 : spsGroundLib/Ground  LConnTagsString=a
  Series RLC Branch : spsSeriesRLCBranchLib/Series RLC Branch  LConnTagsString=__new0  RConnTagsString=__new0  BranchType=C  Resistance=1  Inductance=1e-3  SetiL0=off  InitialCurrent=0  Capacitance=c/2*D  Setx0=off  InitialVoltage=0  Measurements=None
  Series RLC Branch1 : spsSeriesRLCBranchLib/Series RLC Branch  LConnTagsString=__new0  RConnTagsString=__new0  BranchType=RL  Resistance=r*D  Inductance=l*D  SetiL0=off  InitialCurrent=0  Capacitance=1e-6  Setx0=off  InitialVoltage=0  Measurements=None
  Series RLC Branch2 : spsSeriesRLCBranchLib/Series RLC Branch  LConnTagsString=__new0  RConnTagsString=__new0  BranchType=C  Resistance=1  Inductance=1e-3  SetiL0=off  InitialCurrent=0  Capacitance=c/2*D  Setx0=off  InitialVoltage=0  Measurements=None
  Conn1 : PMIOPort  Side=Left
  Conn2 : PMIOPort  Port=2  Side=Right
  connections:
  Series RLC Branch/LConn1 -- Conn1/RConn1 -- Series RLC Branch1/RConn1
  Ground1/LConn1 -- Series RLC Branch2/RConn1
  Ground/LConn1 -- Series RLC Branch/RConn1
  Series RLC Branch1/LConn1 -- Conn2/RConn1 -- Series RLC Branch2/LConn1

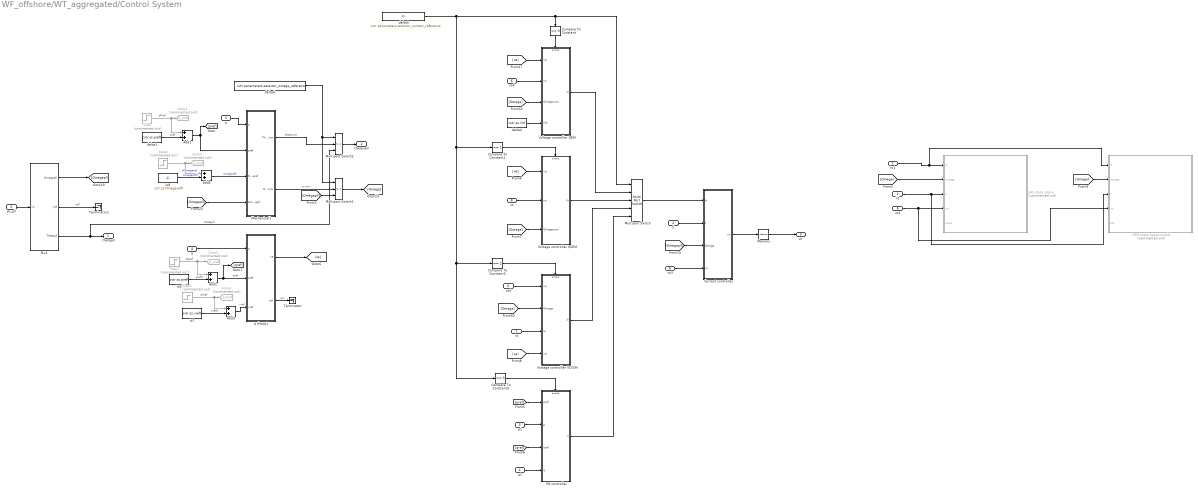
== system WF_offshore/WT_aggregated/Control System ==
  io : Inport
  il : Inport  Port=2
  p : Inport  Port=3
  q : Inport  Port=4
  vo_pll : Inport  Port=5
  vo : Inport  Port=6
  Add{1..4} (4 alike) : Sum
  Compare To Constant : simulink/Logic and Bit Operations/Compare To Constant  relop===  const=0  OutDataTypeStr=boolean
  Compare To Constant1 : simulink/Logic and Bit Operations/Compare To Constant  relop===  const=1  OutDataTypeStr=boolean
  Compare To Constant2 : simulink/Logic and Bit Operations/Compare To Constant  relop===  const=2  OutDataTypeStr=boolean
  Compare To Constant3 : simulink/Logic and Bit Operations/Compare To Constant  relop===  const=3  OutDataTypeStr=boolean
  Current controller : Subsystem
  GFL state space : Subsystem  Commented=on
  GFM State Space model : Subsystem  Commented=on
  Goto2 : Goto  Commented=on  GotoTag=d_pref  TagVisibility=global
  Goto3 : Goto  Commented=on  GotoTag=d_qref  TagVisibility=global
  Goto4 : Goto  Commented=on  GotoTag=d_Oref  TagVisibility=global
  Goto6 : Goto  Commented=on  GotoTag=d_Vref  TagVisibility=global
  Mechanical1 : Subsystem
  Memory : Memory  InitialCondition=cvtr.ss.vir0
  Multiport Switch : MultiPortSwitch  DataPortOrder=Zero-based contiguous  Inputs=4  zeroidx=on  SaturateOnIntegerOverflow=off  InputSameDT=off
  Multiport Switch1 : MultiPortSwitch  DataPortOrder=Zero-based contiguous  Inputs=2  zeroidx=on  SaturateOnIntegerOverflow=off  InputSameDT=off
  Multiport Switch2 : MultiPortSwitch  DataPortOrder=Zero-based contiguous  Inputs=2  zeroidx=on  SaturateOnIntegerOverflow=off  InputSameDT=off
  PLL1 : Subsystem
  PQ controller : Subsystem
  Step : Step  Commented=on  Time=2  After=-0.05  SampleTime=0
  Step1 : Step  Commented=on  Time=1.5  After=0.03  SampleTime=0
  Step2 : Step  Commented=on  Time=2  After=0.001  SampleTime=0
  Step3 : Step  Commented=on  Time=2  After=0.001  SampleTime=0
  Terminator : Terminator
  Terminator1 : Terminator
  Voltage controller DEM : Subsystem
  Voltage controller QSEM : Subsystem
  Voltage controller VCVSM : Subsystem
  delta1 : Constant  Value=cvtr.ss.pref0
  delta4 : Constant  Value=cvtr.ss.ilr0
  delta5 : Constant  Value=cvtr.parameters.selector_current_reference
  delta6 : Constant  Value=cvtr.parameters.selector_omega_reference
  il1 : InportShadow  Port=2
  io1 : InportShadow
  io6 : Constant  Value=cvtr.ss.qref0
  io7 : Constant  Value=cvtr.ss.vref0
  io8 : Constant  Value=cvtr.ss.Omegaref0
  p1 : InportShadow  Port=3
  q droop1 : Subsystem
  q1 : InportShadow  Port=4
  vo{1,3..5} (4 alike) : InportShadow  Port=6
  thetapll : Outport
  thetavsm : Outport  Port=2
  vir : Outport  Port=3
  wires:
  Voltage controller DEM/1(ilr) -> Multiport Switch/2
  Add1/1 -> [pref], Mechanical1/2(pref)
  delta4/1 -> Voltage controller DEM/4(ilr0)
  Multiport Switch/1 -> Current controller/1(ilr)
  Add2/1 -> [qref], q droop1/2(qref)  "qref"
  delta1/1 -> Add1/2  "pref"
  q droop1/2(qm) -> Terminator/1  "qm"
  Add4/1 -> Mechanical1/3(Omegaref)  "omegaref"
  io7/1 -> Add3/2  "vref0"
  [Omega] -> Voltage controller QSEM/3(Omegavsm)
  io8/1 -> Add4/2  "omegaref0"
  Step/1 -> Add1/1, Goto2/1  "dPref"
  [ve] -> Voltage controller QSEM/1(ve)
  delta5/1 -> Compare To Constant3/1, Compare To Constant2/1, Compare To Constant1/1, Multiport Switch/1, Compare To Constant/1
  io6/1 -> Add2/2  "qref0"
  Add3/1 -> q droop1/3(vref)  "vref"
  q/1 -> q droop1/1(q)
  [Omega] -> Voltage controller VCVSM/2(Omega)
  [ve] -> Voltage controller DEM/1(ve)
  [Omegapll] -> Mechanical1/4(Omegapll)
  [Omega] -> Voltage controller DEM/3(Omegavsm)
  p/1 -> Mechanical1/1(p)
  Voltage controller VCVSM/1(ilr) -> Multiport Switch/4
  vo/1 -> Voltage controller QSEM/2(vo)
  vo_pll/1 -> PLL1/1(vo)
  PLL1/2(vpll) -> Terminator1/1  "vpll"
  q droop1/1(ve) -> [ve]
  Voltage controller QSEM/1(ilr) -> Multiport Switch/3
  Memory/1 -> vir/1
  Current controller/1(vir) -> Memory/1
  p1/1 -> PQ controller/2(p)
  q1/1 -> PQ controller/4(q)
  PQ controller/1(ir) -> Multiport Switch/5
  il/1 -> Current controller/2(il)
  delta6/1 -> Multiport Switch2/1, Multiport Switch1/1
  [Omegapll] -> Current controller/3(Omega)
  Mechanical1/2(Omegavsm) -> Multiport Switch1/2  "wvsm"
  [Omegapll] -> Multiport Switch1/3
  Multiport Switch2/1 -> thetavsm/1
  Mechanical1/1(Thetavsm) -> Multiport Switch2/2  "thetavsm"
  Compare To Constant/1 -> Voltage controller DEM/Enable
  Compare To Constant1/1 -> Voltage controller QSEM/Enable
  Compare To Constant2/1 -> Voltage controller VCVSM/Enable
  Compare To Constant3/1 -> PQ controller/Enable
  Multiport Switch1/1 -> [Omega]
  PLL1/1(Omegapll) -> [Omegapll]
  PLL1/3(Thetapll) -> Multiport Switch2/3, thetapll/1  "thetapll"
  io/1 -> Voltage controller VCVSM/3(io)
  vo3/1 -> Current controller/4(vo)
  vo4/1 -> Voltage controller DEM/2(vo)
  vo5/1 -> Voltage controller VCVSM/1(vo)
  [ve] -> Voltage controller VCVSM/4(ve)
  [pref] -> PQ controller/1(pref)
  [qref] -> PQ controller/3(qref)
  Step1/1 -> Goto3/1, Add2/1  "dQref"
  Step2/1 -> Add4/1, Goto4/1  "dOmegaref"
  Step3/1 -> Add3/1, Goto6/1  "dVref"
  [Omega] -> GFL state space/2(omega)
  vo1/1 -> GFM State Space model/4(vo), GFL state space/4(vo)
  il1/1 -> GFM State Space model/3(il), GFL state space/3(il)
  io1/1 -> GFM State Space model/1(io), GFL state space/1(io)
  [Omega] -> GFM State Space model/2(omega)

== system WF_offshore/WT_aggregated/Inverse Park1 ==
  x_dq : Inport
  delta : Inport  Port=2
  Demux1 : Demux  Outputs=2
  Fcn : Fcn  Expr=cos(u(3))*u(1)-sin(u(3))*u(2)
  Fcn1 : Fcn  Expr=cos(u(3)-2/3*pi)*u(1)-sin(u(3)-2/3*pi)*u(2)
  Fcn2 : Fcn  Expr=cos(u(3)+2/3*pi)*u(1)-sin(u(3)+2/3*pi)*u(2)
  Mux : Mux  Inputs=3
  Mux1 : Mux  Inputs=3
  x_abc : Outport
  wires:
  Mux/1 -> Fcn1/1, Fcn2/1, Fcn/1
  Demux1/2 -> Mux/2
  Demux1/1 -> Mux/1
  Fcn/1 -> Mux1/1
  Fcn1/1 -> Mux1/2
  Fcn2/1 -> Mux1/3
  Mux1/1 -> x_abc/1
  x_dq/1 -> Demux1/1
  delta/1 -> Mux/3

== system WF_offshore/WT_aggregated/Subsystem1 ==
  v_abc : Inport
  Controlled Voltage Source : spsControlledVoltageSourceLib/Controlled Voltage Source  Initialize=on  Source_Type=AC  Amplitude=0  Phase=0  Frequency=0  Measurements=None
  Controlled Voltage Source1 : spsControlledVoltageSourceLib/Controlled Voltage Source  Initialize=on  Source_Type=AC  Amplitude=0  Phase=0  Frequency=0  Measurements=None
  Controlled Voltage Source2 : spsControlledVoltageSourceLib/Controlled Voltage Source  Initialize=on  Source_Type=AC  Amplitude=0  Phase=0  Frequency=0  Measurements=None
  Demux : Demux  Outputs=3
  Ground : spsGroundLib/Ground  LConnTagsString=a
  va1 : PMIOPort  Side=Right
  vb1 : PMIOPort  Port=2  Side=Right
  vc1 : PMIOPort  Port=3  Side=Right
  wires:
  v_abc/1 -> Demux/1
  Demux/3 -> Controlled Voltage Source2/1
  Demux/2 -> Controlled Voltage Source1/1
  Demux/1 -> Controlled Voltage Source/1
  connections:
  Controlled Voltage Source/LConn1 -- Controlled Voltage Source1/LConn1 -- Controlled Voltage Source2/LConn1 -- Ground/LConn1
  vc1/RConn1 -- Controlled Voltage Source2/RConn1
  vb1/RConn1 -- Controlled Voltage Source1/RConn1
  va1/RConn1 -- Controlled Voltage Source/RConn1

== system WF_offshore/WT_aggregated/Subsystem6 ==
  x_d+ix_q : Inport
  Complex to Real-Imag2 : ComplexToRealImag
  Mux : Mux  Inputs=2
  x_dq : Outport
  wires:
  Complex to Real-Imag2/1 -> Mux/1
  Complex to Real-Imag2/2 -> Mux/2
  Mux/1 -> x_dq/1
  x_d+ix_q/1 -> Complex to Real-Imag2/1

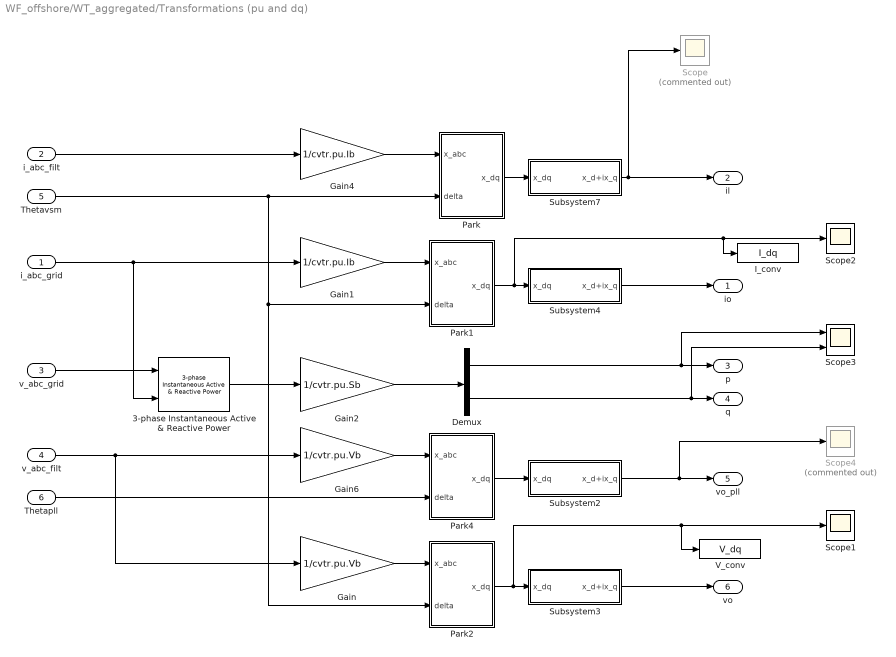
== system WF_offshore/WT_aggregated/Transformations (pu and dq) ==
  i_abc_grid : Inport
  i_abc_filt : Inport  Port=2
  v_abc_grid : Inport  Port=3
  v_abc_filt : Inport  Port=4
  Thetavsm : Inport  Port=5
  Thetapll : Inport  Port=6
  3-phase Instantaneous Active & Reactive Power : powerlib_extras/Measurements/3-phase  Instantaneous  Active & Reactive Power
  Demux : Demux  Outputs=2
  Gain : Gain  Gain=1/cvtr.pu.Vb
  Gain1 : Gain  Gain=1/cvtr.pu.Ib
  Gain2 : Gain  Gain=1/cvtr.pu.Sb
  Gain4 : Gain  Gain=1/cvtr.pu.Ib
  Gain6 : Gain  Gain=1/cvtr.pu.Vb
  I_conv : ToWorkspace  VariableName=I_dq  SaveFormat=Structure With Time  SampleTime=-1
      settings: MaxDataPoints=1000000
  Park : Subsystem
  Park1 : Subsystem
  Park2 : Subsystem
  Park4 : Subsystem
  Scope : Scope  Commented=on
  Scope1 : Scope
  Scope2 : Scope
  Scope3 : Scope  NumInputPorts=2
  Scope4 : Scope  Commented=on
  Subsystem2 : Subsystem
  Subsystem3 : Subsystem
  Subsystem4 : Subsystem
  Subsystem7 : Subsystem
  V_conv : ToWorkspace  VariableName=V_dq  SaveFormat=Structure With Time  SampleTime=-1
      settings: MaxDataPoints=1000000
  io : Outport
  il : Outport  Port=2
  p : Outport  Port=3
  q : Outport  Port=4
  vo_pll : Outport  Port=5
  vo : Outport  Port=6
  wires:
  Gain6/1 -> Park4/1(x_abc)
  i_abc_grid/1 -> 3-phase Instantaneous Active & Reactive Power/2, Gain1/1
  Gain2/1 -> Demux/1
  Gain1/1 -> Park1/1(x_abc)
  Gain/1 -> Park2/1(x_abc)
  Gain4/1 -> Park/1(x_abc)
  Park4/1(x_dq) -> Subsystem2/1(x_dq)
  Demux/1 -> Scope3/1, p/1
  i_abc_filt/1 -> Gain4/1
  Thetapll/1 -> Park4/2(delta)
  Subsystem2/1(x_d+ix_q) -> Scope4/1, vo_pll/1
  Thetavsm/1 -> Park1/2(delta), Park2/2(delta), Park/2(delta)
  Demux/2 -> Scope3/2, q/1
  v_abc_grid/1 -> 3-phase Instantaneous Active & Reactive Power/1
  3-phase Instantaneous Active & Reactive Power/1 -> Gain2/1
  Subsystem4/1(x_d+ix_q) -> io/1
  Subsystem7/1(x_d+ix_q) -> il/1, Scope/1
  Subsystem3/1(x_d+ix_q) -> vo/1
  Park/1(x_dq) -> Subsystem7/1(x_dq)
  Park1/1(x_dq) -> I_conv/1, Scope2/1, Subsystem4/1(x_dq)
  Park2/1(x_dq) -> V_conv/1, Scope1/1, Subsystem3/1(x_dq)
  v_abc_filt/1 -> Gain/1, Gain6/1

== system WF_offshore/WT_aggregated/filter capacitance1 ==
  Ground : spsGroundLib/Ground  LConnTagsString=a
  Series RLC Branch : spsSeriesRLCBranchLib/Series RLC Branch  LConnTagsString=__new0  RConnTagsString=__new0  BranchType=C  Resistance=R  Inductance=L  SetiL0=on  InitialCurrent=ia0  Capacitance=cvtr.parameters.Cf  Setx0=on  InitialVoltage=cvtr.ss.vo0a  Measurements=None
  Series RLC Branch1 : spsSeriesRLCBranchLib/Series RLC Branch  LConnTagsString=__new0  RConnTagsString=__new0  BranchType=C  Resistance=R  Inductance=L  SetiL0=on  InitialCurrent=ia0  Capacitance=cvtr.parameters.Cf  Setx0=on  InitialVoltage=cvtr.ss.vo0b  Measurements=None
  Series RLC Branch2 : spsSeriesRLCBranchLib/Series RLC Branch  LConnTagsString=__new0  RConnTagsString=__new0  BranchType=C  Resistance=R  Inductance=L  SetiL0=on  InitialCurrent=ia0  Capacitance=cvtr.parameters.Cf  Setx0=on  InitialVoltage=cvtr.ss.vo0c  Measurements=None
  Three-Phase V-I Measurement : spsThreePhaseVIMeasurementLib/Three-Phase V-I Measurement  VoltageMeasurement=phase-to-ground  SetLabelV=off  LabelV=Vabc  Vpu=off  VpuLL=off  CurrentMeasurement=no  SetLabelI=off  LabelI=Iabc  Ipu=off  Pbase=100e6  Vbase=500e3  OutputType=Complex  PhasorSimulation=off  PSBequivalent=0
  A : PMIOPort  Side=Left
  B : PMIOPort  Port=2  Side=Left
  C : PMIOPort  Port=3  Side=Left
  v_abc : Outport
  wires:
  Three-Phase V-I Measurement/1 -> v_abc/1
  connections:
  A/RConn1 -- Three-Phase V-I Measurement/LConn1
  B/RConn1 -- Three-Phase V-I Measurement/LConn2
  C/RConn1 -- Three-Phase V-I Measurement/LConn3
  Three-Phase V-I Measurement/RConn1 -- Series RLC Branch/LConn1
  Three-Phase V-I Measurement/RConn2 -- Series RLC Branch1/LConn1
  Three-Phase V-I Measurement/RConn3 -- Series RLC Branch2/LConn1
  Series RLC Branch/RConn1 -- Ground/LConn1 -- Series RLC Branch1/RConn1 -- Series RLC Branch2/RConn1

== system WF_offshore/WT_aggregated/filter inductance1 ==
  Series RLC Branch : spsSeriesRLCBranchLib/Series RLC Branch  LConnTagsString=__new0  RConnTagsString=__new0  BranchType=RL  Resistance=cvtr.parameters.Rf  Inductance=cvtr.parameters.Lf  SetiL0=on  InitialCurrent=cvtr.ss.il0a  Capacitance=1e-6  Setx0=off  InitialVoltage=0  Measurements=None
  Series RLC Branch1 : spsSeriesRLCBranchLib/Series RLC Branch  LConnTagsString=__new0  RConnTagsString=__new0  BranchType=RL  Resistance=cvtr.parameters.Rf  Inductance=cvtr.parameters.Lf  SetiL0=on  InitialCurrent=cvtr.ss.il0b  Capacitance=1e-6  Setx0=off  InitialVoltage=0  Measurements=None
  Series RLC Branch2 : spsSeriesRLCBranchLib/Series RLC Branch  LConnTagsString=__new0  RConnTagsString=__new0  BranchType=RL  Resistance=cvtr.parameters.Rf  Inductance=cvtr.parameters.Lf  SetiL0=on  InitialCurrent=cvtr.ss.il0c  Capacitance=1e-6  Setx0=off  InitialVoltage=0  Measurements=None
  Three-Phase V-I Measurement : spsThreePhaseVIMeasurementLib/Three-Phase V-I Measurement  VoltageMeasurement=no  SetLabelV=off  LabelV=Vabc  Vpu=off  VpuLL=off  CurrentMeasurement=yes  SetLabelI=off  LabelI=Iabc  Ipu=off  Pbase=100e6  Vbase=500e3  OutputType=Complex  PhasorSimulation=off  PSBequivalent=0
  A : PMIOPort  Side=Left
  B : PMIOPort  Port=2  Side=Left
  C : PMIOPort  Port=3  Side=Left
  a : PMIOPort  Port=4  Side=Right
  b : PMIOPort  Port=5  Side=Right
  c : PMIOPort  Port=6  Side=Right
  i_abc : Outport
  wires:
  Three-Phase V-I Measurement/1 -> i_abc/1
  connections:
  c/RConn1 -- Three-Phase V-I Measurement/RConn3
  C/RConn1 -- Series RLC Branch2/LConn1
  b/RConn1 -- Three-Phase V-I Measurement/RConn2
  B/RConn1 -- Series RLC Branch1/LConn1
  a/RConn1 -- Three-Phase V-I Measurement/RConn1
  A/RConn1 -- Series RLC Branch/LConn1
  Series RLC Branch2/RConn1 -- Three-Phase V-I Measurement/LConn3
  Series RLC Branch1/RConn1 -- Three-Phase V-I Measurement/LConn2
  Series RLC Branch/RConn1 -- Three-Phase V-I Measurement/LConn1

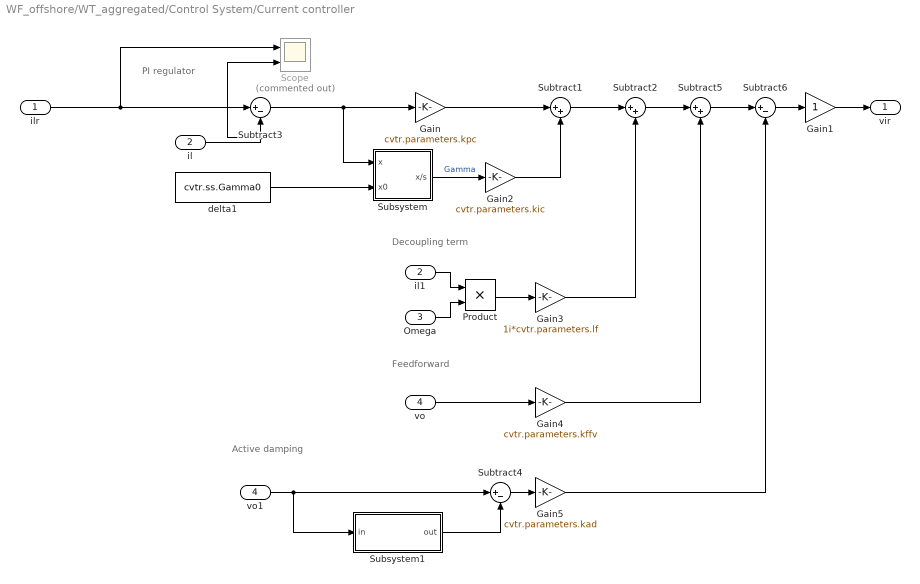
== system WF_offshore/WT_aggregated/Control System/Current controller ==
  note: Active damping
  note: Feedforward
  note: Decoupling term
  note: PI regulator
  ilr : Inport
  il : Inport  Port=2
  Omega : Inport  Port=3
  vo : Inport  Port=4
  Gain : Gain  Gain=cvtr.parameters.kpc
  Gain1 : Gain
  Gain2 : Gain  Gain=cvtr.parameters.kic
  Gain3 : Gain  Gain=1i*cvtr.parameters.lf
  Gain4 : Gain  Gain=cvtr.parameters.kffv
  Gain5 : Gain  Gain=cvtr.parameters.kad
  Product : Product  RndMeth=Zero
  Scope : Scope  Commented=on  NumInputPorts=2
  Subsystem : Subsystem
  Subsystem1 : Subsystem  mask{Omega=cvtr.parameters.Omegaad, xd0=cvtr.ss.Phid0, xq0=cvtr.ss.Phiq0}
  Subtract1 : Sum  Inputs=|++
  Subtract2 : Sum  Inputs=|++
  Subtract3 : Sum  Inputs=|+-
  Subtract4 : Sum  Inputs=|+-
  Subtract5 : Sum  Inputs=|++
  Subtract6 : Sum  Inputs=|+-
  delta1 : Constant  Value=cvtr.ss.Gamma0
  il1 : InportShadow  Port=2
  vo1 : InportShadow  Port=4
  vir : Outport
  wires:
  Gain2/1 -> Subtract1/2
  Gain3/1 -> Subtract2/2
  Product/1 -> Gain3/1
  Omega/1 -> Product/2
  vo/1 -> Gain4/1
  Gain4/1 -> Subtract5/2
  Gain5/1 -> Subtract6/2
  Subtract4/1 -> Gain5/1
  delta1/1 -> Subsystem/2(x0)
  il/1 -> Scope/2, Subtract3/2
  Subsystem/1(x/s) -> Gain2/1  "Gamma"
  il1/1 -> Product/1
  Subtract1/1 -> Subtract2/1
  vo1/1 -> Subsystem1/1(in), Subtract4/1
  Subsystem1/1(out) -> Subtract4/2
  Subtract2/1 -> Subtract5/1
  Subtract5/1 -> Subtract6/1
  Gain/1 -> Subtract1/1
  Subtract6/1 -> Gain1/1
  Gain1/1 -> vir/1
  Subtract3/1 -> Subsystem/1(x), Gain/1
  ilr/1 -> Scope/1, Subtract3/1

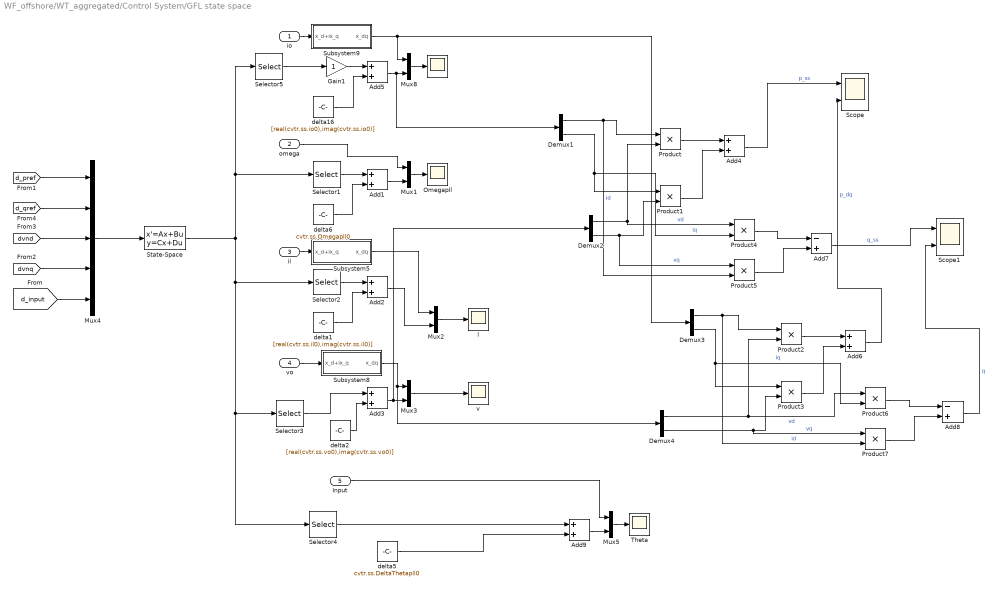
== system WF_offshore/WT_aggregated/Control System/GFL state space ==
  io : Inport
  omega : Inport  Port=2
  il : Inport  Port=3
  vo : Inport  Port=4
  Input : Inport  Port=5
  " " : Scope
  " l" : Scope
  Add{1..6,9} (7 alike) : Sum
  Add7 : Sum  Inputs=-+
  Add8 : Sum  Inputs=-+
  Demux{1..4} (4 alike) : Demux  Outputs=2
  Gain1 : Gain
  Mux{1..3,5,8} (5 alike) : Mux  Inputs=2
  Mux4 : Mux  Inputs=5
  Omegapll : Scope
  Product{,1..7} (8 alike) : Product
  Scope : Scope  NumInputPorts=2
  Scope1 : Scope  NumInputPorts=2
  Selector1 : Selector  IndexOptions=Index vector (dialog)  Indices=15  OutputSizes=1
  Selector2 : Selector  IndexOptions=Index vector (dialog)  Indices=[1,2]  OutputSizes=1
  Selector3 : Selector  IndexOptions=Index vector (dialog)  Indices=[3,4]  OutputSizes=1
  Selector4 : Selector  IndexOptions=Index vector (dialog)  Indices=16  OutputSizes=1
  Selector5 : Selector  IndexOptions=Index vector (dialog)  Indices=[5,6]  OutputSizes=1
  State-Space : StateSpace  A=cvtr.A  B=cvtr.B  C=eye(size(cvtr.A))  D=zeros(size(cvtr.B))  InitialCondition=0
  Subsystem5 : Subsystem
  Subsystem8 : Subsystem
  Subsystem9 : Subsystem
  Theta : Scope
  delta1 : Constant  Value=[real(cvtr.ss.il0),imag(cvtr.ss.il0)]
  delta16 : Constant  Value=[real(cvtr.ss.io0),imag(cvtr.ss.io0)]
  delta2 : Constant  Value=[real(cvtr.ss.vo0),imag(cvtr.ss.vo0)]
  delta5 : Constant  Value=cvtr.ss.DeltaThetapll0
  delta6 : Constant  Value=cvtr.ss.Omegapll0
  v : Scope
  wires:
  io/1 -> Subsystem9/1(x_d+ix_q)
  delta6/1 -> Add1/2
  Add5/1 -> Demux1/1, Mux8/2
  Mux1/1 -> Omegapll/1
  Mux2/1 -> " l"/1
  Mux3/1 -> v/1
  omega/1 -> Mux1/1
  delta1/1 -> Add2/2
  Add3/1 -> Demux2/1, Mux3/2
  delta2/1 -> Add3/2
  Selector5/1 -> Gain1/1
  Mux8/1 -> " "/1
  Add1/1 -> Mux1/2
  vo/1 -> Subsystem8/1(x_d+ix_q)
  il/1 -> Subsystem5/1(x_d+ix_q)
  Add2/1 -> Mux2/2
  delta16/1 -> Add5/2
  Selector2/1 -> Add2/1
  Selector1/1 -> Add1/1
  State-Space/1 -> Selector5/1, Selector1/1, Selector3/1, Selector4/1, Selector2/1
  Subsystem5/1(x_dq) -> Mux2/1
  Mux4/1 -> State-Space/1
  Demux1/1 -> Product5/2, Product/1  "id"
  Demux2/1 -> Product4/1, Product/2  "vd"
  Demux1/2 -> Product4/2, Product1/1  "iq"
  Demux2/2 -> Product5/1, Product1/2  "vq"
  Product/1 -> Add4/1
  Product1/1 -> Add4/2
  Add4/1 -> Scope/1  "p_ss"
  Product3/1 -> Add6/2
  Product2/1 -> Add6/1
  Demux4/2 -> Product7/1, Product3/2  "vq"
  Demux3/2 -> Product6/2, Product3/1  "iq"
  Demux4/1 -> Product2/2, Product6/1  "vd"
  Demux3/1 -> Product7/2, Product2/1  "id"
  Subsystem8/1(x_dq) -> Demux4/1, Mux3/1
  Subsystem9/1(x_dq) -> Demux3/1, Mux8/1
  Add6/1 -> Scope/2  "p_dq"
  Product4/1 -> Add7/1
  Product5/1 -> Add7/2
  Add7/1 -> Scope1/1  "q_ss"
  Add8/1 -> Scope1/2  "q"
  Product7/1 -> Add8/2
  Product6/1 -> Add8/1
  [d_input] -> Mux4/5
  Gain1/1 -> Add5/1
  Selector3/1 -> Add3/1
  Mux5/1 -> Theta/1
  Add9/1 -> Mux5/2
  delta5/1 -> Add9/2
  Selector4/1 -> Add9/1
  Input/1 -> Mux5/1
  [dvnq] -> Mux4/4
  [dvnd] -> Mux4/3
  [d_pref] -> Mux4/1
  [d_qref] -> Mux4/2

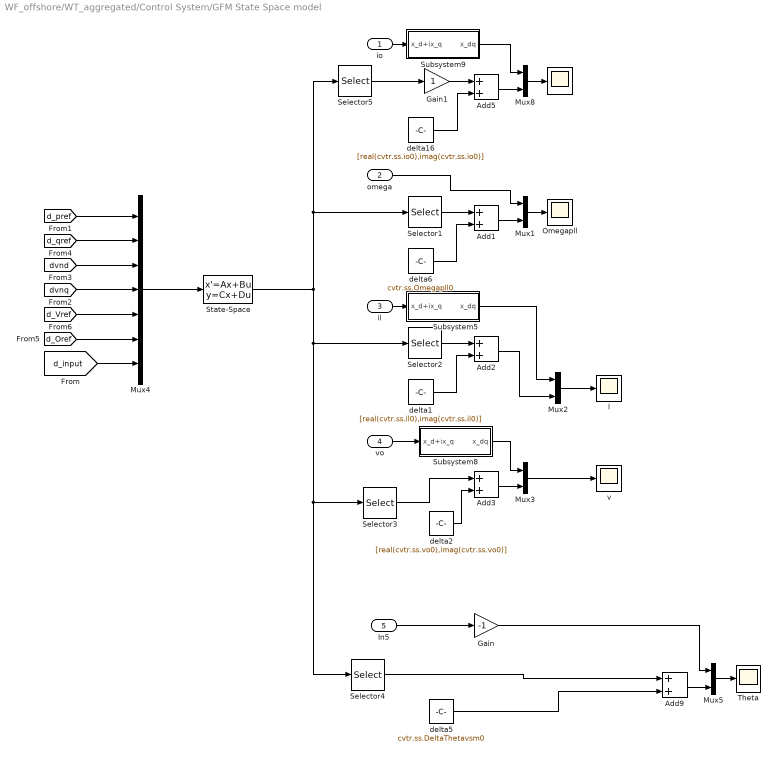
== system WF_offshore/WT_aggregated/Control System/GFM State Space model ==
  io : Inport
  omega : Inport  Port=2
  il : Inport  Port=3
  vo : Inport  Port=4
  In5 : Inport  Port=5
  " " : Scope
  " l" : Scope
  Add{1..3,5,9} (5 alike) : Sum
  Gain : Gain  Gain=-1
  Gain1 : Gain
  Mux{1..3,5,8} (5 alike) : Mux  Inputs=2
  Mux4 : Mux  Inputs=7
  Omegapll : Scope
  Selector1 : Selector  IndexOptions=Index vector (dialog)  Indices=12  OutputSizes=1
  Selector2 : Selector  IndexOptions=Index vector (dialog)  Indices=[1,2]  OutputSizes=1
  Selector3 : Selector  IndexOptions=Index vector (dialog)  Indices=[3,4]  OutputSizes=1
  Selector4 : Selector  IndexOptions=Index vector (dialog)  Indices=13  OutputSizes=1
  Selector5 : Selector  IndexOptions=Index vector (dialog)  Indices=[5,6]  OutputSizes=1
  State-Space : StateSpace  A=cvtr.A  B=cvtr.B  C=eye(size(cvtr.A))  D=zeros(size(cvtr.B))  InitialCondition=0
  Subsystem5 : Subsystem
  Subsystem8 : Subsystem
  Subsystem9 : Subsystem
  Theta : Scope
  delta1 : Constant  Value=[real(cvtr.ss.il0),imag(cvtr.ss.il0)]
  delta16 : Constant  Value=[real(cvtr.ss.io0),imag(cvtr.ss.io0)]
  delta2 : Constant  Value=[real(cvtr.ss.vo0),imag(cvtr.ss.vo0)]
  delta5 : Constant  Value=cvtr.ss.DeltaThetavsm0
  delta6 : Constant  Value=cvtr.ss.Omegapll0
  v : Scope
  wires:
  [dvnd] -> Mux4/3
  [dvnq] -> Mux4/4
  Selector3/1 -> Add3/1
  Gain1/1 -> Add5/1
  [d_input] -> Mux4/7
  Subsystem9/1(x_dq) -> Mux8/1
  Subsystem8/1(x_dq) -> Mux3/1
  Mux4/1 -> State-Space/1
  Subsystem5/1(x_dq) -> Mux2/1
  State-Space/1 -> Selector2/1, Selector3/1, Selector4/1, Selector1/1, Selector5/1
  Selector1/1 -> Add1/1
  Selector2/1 -> Add2/1
  delta16/1 -> Add5/2
  Add2/1 -> Mux2/2
  il/1 -> Subsystem5/1(x_d+ix_q)
  vo/1 -> Subsystem8/1(x_d+ix_q)
  Add1/1 -> Mux1/2
  Mux8/1 -> " "/1
  Selector5/1 -> Gain1/1
  delta2/1 -> Add3/2
  Add3/1 -> Mux3/2
  delta1/1 -> Add2/2
  omega/1 -> Mux1/1
  Mux3/1 -> v/1
  Mux2/1 -> " l"/1
  Mux1/1 -> Omegapll/1
  Add5/1 -> Mux8/2
  delta6/1 -> Add1/2
  io/1 -> Subsystem9/1(x_d+ix_q)
  [d_pref] -> Mux4/1
  [d_qref] -> Mux4/2
  [d_Vref] -> Mux4/5
  [d_Oref] -> Mux4/6
  In5/1 -> Gain/1
  Selector4/1 -> Add9/1
  Add9/1 -> Mux5/2
  Mux5/1 -> Theta/1
  delta5/1 -> Add9/2
  Gain/1 -> Mux5/1

== system WF_offshore/WT_aggregated/Control System/Mechanical1 ==
  p : Inport
  pref : Inport  Port=2
  Omegaref : Inport  Port=3
  Omegapll : Inport  Port=4
  Constant : Constant  Value=cvtr.parameters.enable_pll
  Gain : Gain  Gain=1/cvtr.parameters.ta
  Gain1 : Gain  Gain=cvtr.parameters.kd
  Gain2 : Gain  Gain=cvtr.parameters.kdrpOmega
  Gain3 : Gain  Gain=cvtr.pu.Omegab
  Integrator1 : Integrator  InitialConditionSource=external
  Integrator2 : Integrator  InitialConditionSource=external
  Subtract : Sum  Inputs=-+--
  Subtract1 : Sum  Inputs=-+
  Subtract2 : Sum  Inputs=-+
  Switch : Switch  Criteria=u2 > Threshold  SaturateOnIntegerOverflow=off  InputSameDT=off
  Transfer Fcn (with initial outputs) : simulink_extras/Additional Linear/Transfer Fcn (with initial outputs)  N=[cvtr.parameters.Omegadf]  D="[1  cvtr.parameters.Omegadf]"  Y0=cvtr.ss.Kappa0  U0=cvtr.ss.Kappa0
  delta2 : Constant  Value=cvtr.ss.DeltaThetavsm_mech0
  io5 : Constant  Value=cvtr.ss.Omegavsm0
  Thetavsm : Outport
  Omegavsm : Outport  Port=2
  wires:
  p/1 -> Subtract/1
  pref/1 -> Subtract/2
  Subtract/1 -> Gain/1
  Gain1/1 -> Subtract/3
  Subtract1/1 -> Gain1/1
  io5/1 -> Integrator2/2
  Gain/1 -> Integrator2/1
  Omegaref/1 -> Subtract2/1
  Subtract2/1 -> Gain2/1
  Gain2/1 -> Subtract/4
  Gain3/1 -> Integrator1/1
  Omegapll/1 -> Switch/1
  Constant/1 -> Switch/2
  Transfer Fcn (with initial outputs)/1 -> Switch/3
  Integrator2/1 -> Gain3/1, Transfer Fcn (with initial outputs)/1, Subtract2/2, Subtract1/2, Omegavsm/1
  Switch/1 -> Subtract1/1
  Integrator1/1 -> Thetavsm/1
  delta2/1 -> Integrator1/2
